simulink model "PM_simple_19b"  (R2019b)
settings: Solver=FixedStepAuto  StartTime=0.0  StopTime=inf  RelTol=1e-3  EnableMultiTasking=on
libraries: raspberrypiCommlib x1
settings Model: SimulationMode=external  ExtModeTrigDuration=2  Creator=arekbrodowski  LastModifiedBy=arekbrodowski
settings SolverCC: PositivePriorityOrder=on  AutoInsertRateTranBlk=on
settings DataIOCC: ReturnWorkspaceOutputs=off
settings OptimizationCC: MaxStackSize=64
settings DebuggingCC: ParameterTunabilityLossMsg=error  ArithmeticOperatorsInVariantConditions=warning
settings HardwareCC: ProdBitPerPointer=32  ProdBitPerSizeT=32  ProdBitPerPtrDiffT=32  ProdLargestAtomicInteger=Long  ProdLargestAtomicFloat=Double  ProdWordSize=32  ProdHWDeviceType=ARM Compatible->ARM Cortex  UseEmbeddedCoderFeatures=off
settings SFSimCC: SimUseLocalCustomCode=off  CustomCodeUndefinedFunction=UseInterfaceOnly
settings RTWCC: SystemTargetFile=ert.tlc  HardwareBoard=Raspberry Pi  TLCOptions="-aInlineSetEventsForThisBaseRateFcn=TLC_FALSE -aSuppressMultiTaskScheduler=TLC_FALSE  -aRateBasedStepFcn=0"  TemplateMakefile=ert_default_tmf  GenerateReport=on  RTWUseLocalCustomCode=off  Toolchain=GNU GCC Embedded Linux  BuildConfiguration=Faster Runs  LaunchReport=on
settings CodeAppCC: ForceParamTrailComments=on  OperatorAnnotations=on  StateflowObjectComments=on  MATLABSourceComments=on
settings ERTTargetCC: ERTCustomFileBanners=off  SupportContinuousTime=on  SupportNonInlinedSFcns=on  RemoveResetFunc=off  SupportVariableSizeSignals=on  ModelStepFunctionPrototypeControlCompliant=off  ExtMode=on  ExtModeMexArgs='172.20.10.2' 0 17725  ERTSrcFileBannerTemplate=codertarget_code_template.cgt  ERTHdrFileBannerTemplate=codertarget_code_template.cgt  ERTDataSrcFileTemplate=codertarget_code_template.cgt  ERTDataHdrFileTemplate=codertarget_code_template.cgt

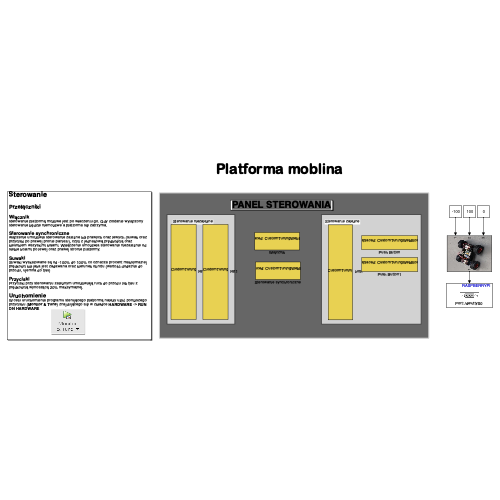
[thumbnail: Simulink's stored preview of the top-level diagram]
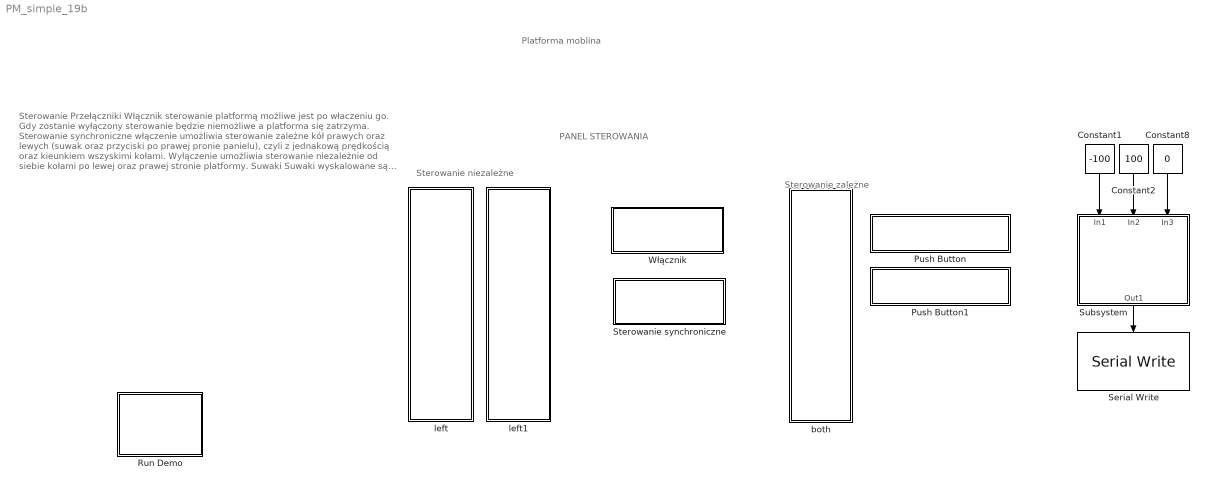
== system PM_simple_19b ==
  note: PANEL STEROWANIA
  note: Sterowanie niezależne
  note: Sterowanie
      |
      | Przełączniki
      |
      | Włącznik
      | sterowanie platformą możliwe jest po właczeniu go. Gdy zostanie wyłączony sterowanie będzie niemożliwe a platforma się zatrzyma.
      |
      | Sterowanie synchroniczne
      | włączenie umożliwia sterowanie zależne kół prawych oraz lewych (suwak oraz przyciski po prawej pronie panielu), czyli z jednakową prędkością oraz kieunkiem wszyskimi kołami. Wyłączenie umożliwia sterowanie niezależnie od siebie kołami po lewej oraz prawej stronie platformy.
      |
      | Suwaki
      | Suwaki wyskalowane są od -100% do 100% co oznacza procent maksymalnej prędkości kół jaka jest zadawana oraz kierunek obrotu (wartość dodatnia do przodu, ujemna do tyłu)
      |
      | Przyciski
      | Przyciski przy sterowaniu zależnym umożliwiają ruch do przodu lub tyłu z prędkością wynoszącą 20% maksymalnej.
      |
      | Uruchomienie
      | W celu uruchomienia programu sterującego platformą należy użyć poniższego przycisku ( Monitor & Tune ) znajdującego się w zkładce HARDWARE -> RUN ON HARDWARE
  note: Platforma moblina
  note: Sterowanie zależne
  Constant1 : Constant  Value=-100  SampleTime=0.01
  Constant2 : Constant  Value=100  SampleTime=0.01
  Constant8 : Constant  Value=0  SampleTime=0.01
  Push Button : Subsystem  Description=Replaced Block  mask(Replaced Block){}
      mask help: This block has been replaced with an empty subsystem because it used functionality that is unavailable in Simulink R2019b.
      mask Display: fprintf('Replaced: %s\n','CustomTuningWebBlock')
  Push Button1 : Subsystem  Description=Replaced Block  mask(Replaced Block){}
      mask help: This block has been replaced with an empty subsystem because it used functionality that is unavailable in Simulink R2019b.
      mask Display: fprintf('Replaced: %s\n','CustomTuningWebBlock')
  Run Demo : Subsystem  Description=Controls host-side RTDX processing.
      mask Display: pic=imread('raspberrypiMonitorAndTune.png');image(pic);
  Serial Write : raspberrypiCommlib/Serial Write  board=Pi 4 Model B  SCIModule_=/dev/ttyS0  Baudrate_=9600  Parity=None  StopBits_=1  HardwareFlowControl=None  ByteOrder=LittleEndian  OutputStatus=off  blockPlatform=RaspberryPi
      settings: SourceProductBaseCode=RASPPI
  Sterowanie synchroniczne : Subsystem  Description=Replaced Block  mask(Replaced Block){}
      mask help: This block has been replaced with an empty subsystem because it used functionality that is unavailable in Simulink R2019b.
      mask Display: fprintf('Replaced: %s\n','CustomTuningWebBlock')
  Subsystem : Subsystem
      mask DialogControl Control2 Prompt: Controller
      mask Display: image('/Users/arekbrodowski/Downloads/IMG_F711DD2AAD95-1.jpeg'); % Use "Edit Image" on toolstrip to change.
  Włącznik : Subsystem  Description=Replaced Block  mask(Replaced Block){}
      mask help: This block has been replaced with an empty subsystem because it used functionality that is unavailable in Simulink R2019b.
      mask Display: fprintf('Replaced: %s\n','CustomTuningWebBlock')
  both : Subsystem  Description=Replaced Block  mask(Replaced Block){}
      mask help: This block has been replaced with an empty subsystem because it used functionality that is unavailable in Simulink R2019b.
      mask Display: fprintf('Replaced: %s\n','CustomTuningWebBlock')
  left : Subsystem  Description=Replaced Block  mask(Replaced Block){}
      mask help: This block has been replaced with an empty subsystem because it used functionality that is unavailable in Simulink R2019b.
      mask Display: fprintf('Replaced: %s\n','CustomTuningWebBlock')
  left1 : Subsystem  Description=Replaced Block  mask(Replaced Block){}
      mask help: This block has been replaced with an empty subsystem because it used functionality that is unavailable in Simulink R2019b.
      mask Display: fprintf('Replaced: %s\n','CustomTuningWebBlock')
  wires:
  Constant1/1 -> Subsystem/1(In1)
  Constant2/1 -> Subsystem/2(In2)
  Constant8/1 -> Subsystem/3(In3)
  Subsystem/1(Out1) -> Serial Write/1

== system PM_simple_19b/Push Button ==

== system PM_simple_19b/Push Button1 ==

== system PM_simple_19b/Run Demo ==

== system PM_simple_19b/Sterowanie synchroniczne ==

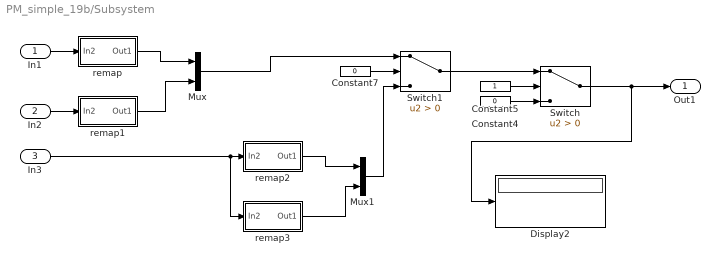
== system PM_simple_19b/Subsystem ==
  In1 : Inport
  In2 : Inport  Port=2
  In3 : Inport  Port=3
  Constant4 : Constant  Value=0  OutDataTypeStr=uint8  SampleTime=1
  Constant5 : Constant  SampleTime=1
  Constant7 : Constant  Value=0  SampleTime=1
  Display2 : Display
  Mux : Mux  Inputs=2
  Mux1 : Mux  Inputs=2
  Switch : Switch  Criteria=u2 > Threshold
  Switch1 : Switch  Criteria=u2 > Threshold
  remap : Subsystem
  remap1 : Subsystem
  remap2 : Subsystem
  remap3 : Subsystem
  Out1 : Outport
  wires:
  Constant7/1 -> Switch1/2
  Mux/1 -> Switch1/1
  In3/1 -> remap3/1(In2), remap2/1(In2)
  Switch/1 -> Out1/1, Display2/1
  remap2/1(Out1) -> Mux1/1
  remap/1(Out1) -> Mux/1
  In2/1 -> remap1/1(In2)
  Mux1/1 -> Switch1/3
  Constant5/1 -> Switch/2
  remap1/1(Out1) -> Mux/2
  Constant4/1 -> Switch/3
  In1/1 -> remap/1(In2)
  remap3/1(Out1) -> Mux1/2
  Switch1/1 -> Switch/1

== system PM_simple_19b/Włącznik ==

== system PM_simple_19b/both ==

== system PM_simple_19b/left ==

== system PM_simple_19b/left1 ==

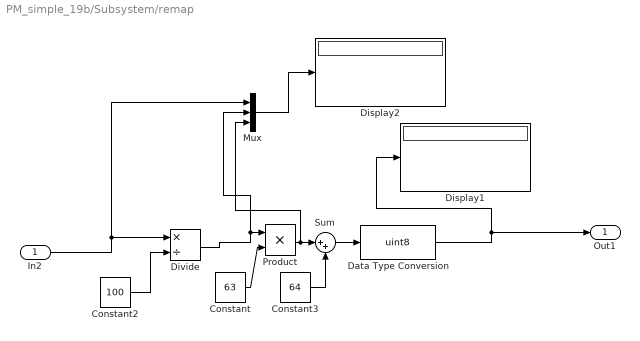
== system PM_simple_19b/Subsystem/remap ==
  In2 : Inport
  Constant : Constant  Value=63
  Constant2 : Constant  Value=100  OutDataTypeStr=double
  Constant3 : Constant  Value=64  OutDataTypeStr=double
  Data Type Conversion : DataTypeConversion  OutDataTypeStr=uint8
  Display1 : Display
  Display2 : Display
  Divide : Product  Inputs=*/
  Mux : Mux  Inputs=3
  Product : Product  OutDataTypeStr=double
  Sum : Sum  Inputs=|++  OutDataTypeStr=double
  Out1 : Outport
  wires:
  Mux/1 -> Display2/1
  Constant2/1 -> Divide/2
  Data Type Conversion/1 -> Out1/1, Display1/1
  Constant/1 -> Product/2
  Product/1 -> Mux/3, Sum/1
  Sum/1 -> Data Type Conversion/1
  Constant3/1 -> Sum/2
  In2/1 -> Divide/1, Mux/1
  Divide/1 -> Mux/2, Product/1

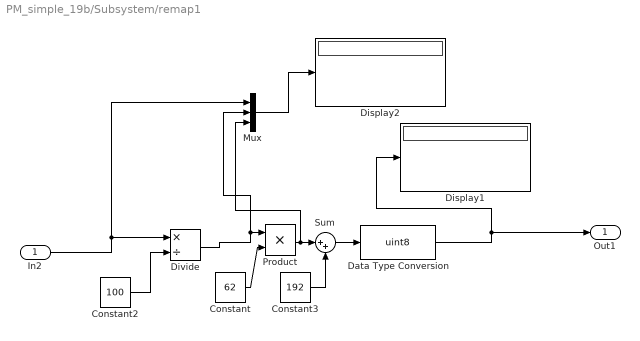
== system PM_simple_19b/Subsystem/remap1 ==
  In2 : Inport
  Constant : Constant  Value=62
  Constant2 : Constant  Value=100  OutDataTypeStr=double
  Constant3 : Constant  Value=192  OutDataTypeStr=double
  Data Type Conversion : DataTypeConversion  OutDataTypeStr=uint8
  Display1 : Display
  Display2 : Display
  Divide : Product  Inputs=*/
  Mux : Mux  Inputs=3
  Product : Product  OutDataTypeStr=double
  Sum : Sum  Inputs=|++  OutDataTypeStr=double
  Out1 : Outport
  wires:
  Mux/1 -> Display2/1
  Constant2/1 -> Divide/2
  Data Type Conversion/1 -> Out1/1, Display1/1
  Constant/1 -> Product/2
  Product/1 -> Mux/3, Sum/1
  Sum/1 -> Data Type Conversion/1
  Constant3/1 -> Sum/2
  In2/1 -> Divide/1, Mux/1
  Divide/1 -> Mux/2, Product/1

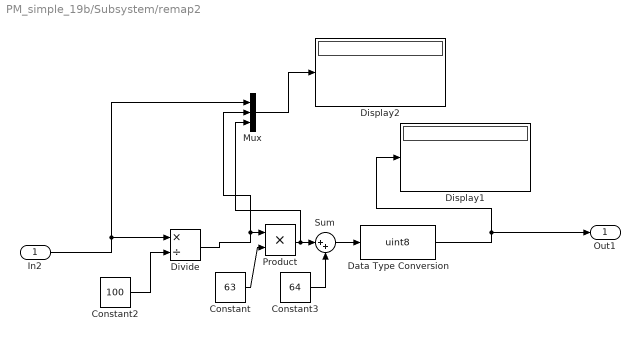
== system PM_simple_19b/Subsystem/remap2 ==
  In2 : Inport
  Constant : Constant  Value=63
  Constant2 : Constant  Value=100  OutDataTypeStr=double
  Constant3 : Constant  Value=64  OutDataTypeStr=double
  Data Type Conversion : DataTypeConversion  OutDataTypeStr=uint8
  Display1 : Display
  Display2 : Display
  Divide : Product  Inputs=*/
  Mux : Mux  Inputs=3
  Product : Product  OutDataTypeStr=double
  Sum : Sum  Inputs=|++  OutDataTypeStr=double
  Out1 : Outport
  wires:
  Mux/1 -> Display2/1
  Constant2/1 -> Divide/2
  Data Type Conversion/1 -> Out1/1, Display1/1
  Constant/1 -> Product/2
  Product/1 -> Mux/3, Sum/1
  Sum/1 -> Data Type Conversion/1
  Constant3/1 -> Sum/2
  In2/1 -> Divide/1, Mux/1
  Divide/1 -> Mux/2, Product/1

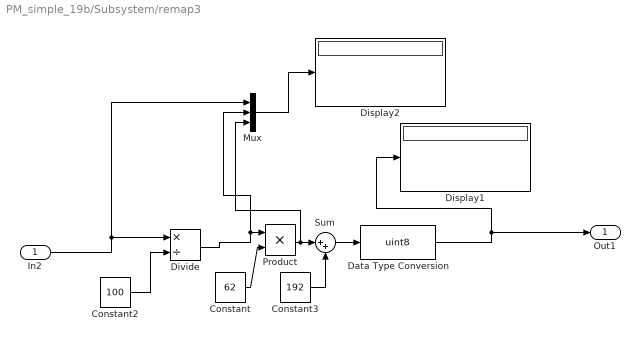
== system PM_simple_19b/Subsystem/remap3 ==
  In2 : Inport
  Constant : Constant  Value=62
  Constant2 : Constant  Value=100  OutDataTypeStr=double
  Constant3 : Constant  Value=192  OutDataTypeStr=double
  Data Type Conversion : DataTypeConversion  OutDataTypeStr=uint8
  Display1 : Display
  Display2 : Display
  Divide : Product  Inputs=*/
  Mux : Mux  Inputs=3
  Product : Product  OutDataTypeStr=double
  Sum : Sum  Inputs=|++  OutDataTypeStr=double
  Out1 : Outport
  wires:
  Mux/1 -> Display2/1
  Constant2/1 -> Divide/2
  Data Type Conversion/1 -> Out1/1, Display1/1
  Constant/1 -> Product/2
  Product/1 -> Mux/3, Sum/1
  Sum/1 -> Data Type Conversion/1
  Constant3/1 -> Sum/2
  In2/1 -> Divide/1, Mux/1
  Divide/1 -> Mux/2, Product/1
